simulink subsystem "Load"  (R2020b)
settings: Solver=VariableStepAuto  StartTime=0.0  StopTime=10.0  RelTol=1e-3
undefined symbols (not defined in the file): DCHigh, DCLow
libraries: nesl_utility x5, fl_lib x5
settings Model: Creator=cao2851  LastModifiedBy=cao2851
settings SimscapeCC: SimscapeNormalizeSystem=off

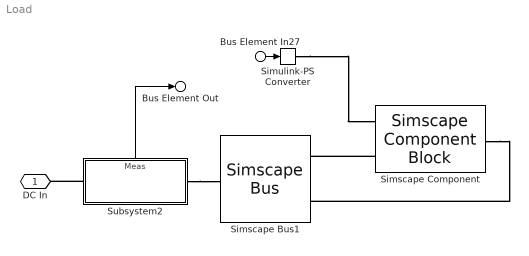
== system Load ==
  Bus Element In27 : Inport  PortName=Ctrl  Element=LoadSetpoint
  Simscape Component : SimscapeComponentBlock  SourceFile=VariablePowerLoad  ComponentPath=VariablePowerLoad  ComponentVariants="[\"VariablePowerLoad\"]"  ComponentVariantNames="[\"VariablePowerLoad\"]"  ClassName=VariablePowerLoad  SchemaVersion=1  Vsoll=350  Slope=100  MinV=0.7  MaxV=1.2  i_specify=off  i_priority=None  i=0 A  i_nominal_specify=off  i_nominal_unit=A  i_nominal_value=1  v_specify=off  v_priority=None  v=0 V  v_nominal_specify=off  v_nominal_unit=V  v_nominal_value=1  Psoll_specify=off  Psoll_priority=None  Psoll=0 W  Psoll_nominal_specify=off  Psoll_nominal_unit=W  Psoll_nominal_value=1
      settings: CopyFcn=simscape.engine.sli.internal.componentblockcallback(gcbh,'COPY')  PreCopyFcn=simscape.engine.sli.internal.componentblockcallback(gcbh,'PRECOPY')  PreDeleteFcn=simscape.engine.sli.internal.componentblockcallback(gcbh,'PREDELETE')  InternalSimscapePortConfiguration="{\"Bottom\":[],\"Left\":[{\"id\":\"Power\",\"label\":\"P\",\"type\":\"input\"},{\"id\":\"p\",\"label\":\"+\",\"type\":\"foundation.electrical.electrical\"}],\"Right\":[{\"id\":\"n\",\"label\":\"-\",\"type\":\"foundation.electrical.electrical\"}],\"Top\":[]}"
      mask Type: Variable power load. It might be necesarry to use local simscape solver.
  Simscape Bus1 : SimscapeBus  HierarchyStrings=DCHigh;DCLow
  Simulink-PS Converter : nesl_utility/Simulink-PS Converter  PhysicalDomain=network_engine_domain  SubClassName=ps_input  LeftPortType=input  RightPortType=output  PseudoPeriodic=off  Frequencies=[]  NoiseDistribution=none  NoiseParameters=[]  Unit=1  AffineConversion=off  FilteringAndDerivatives=provide  SimscapeFilterOrder=1  InputFilterTimeConstant=0.001  UdotUserProvided=0
  Subsystem2 : Subsystem
      settings: PortSchema="{\"entries\":[{\"content\":{\"sides\":[{\"content\":{\"connectorIds\":[\"LConn1\"]},\"type\":\"ConnectorPlacement.EquallySpacedRectSide\",\"uuid\":\"6ceb37b8-2165-4d7d-a6fb-f279e2d82052\"},{\"content\":{\"connectorIds\":[\"RConn1\"],\"side\":\"RIGHT\"},\"type\":\"ConnectorPlacement.EquallySpacedRectSide\",\"uuid\":\"4155948b-55c4-4bcd-990d-59b1d009d707\"},{\"content\":{\"connectorIds\":[\"Out1\"],\"side\":\"TOP\"},\"type\":\"ConnectorPlacement.EquallySpacedRectSide\",\"uuid\":\"00a7b829-f817-4a9f-907b-0b6347f161bc\"},{\"content\":{\"connectorIds\":[],\"side\":\"HIDDEN\"},\"type\":\"ConnectorPlacement.EquallySpacedRectSide\",\"uuid\":\"9dcb8e64-3042-4cb3-a9ae-ca9509bc434a\"}]},\"type\":\"ConnectorPlacement.EquallySpacedConnector\",\"uuid\":\"80bcd14e-b03c-415a-a271-317cb15dab1c\"}],\"packageUris\":[\"http://schema.mathworks.com/mf0/Connector/R2020b\"],\"version\":\"1.0\"}"
  DC In : PMIOPort  Side=Left
  Bus Element Out : Outport  PortName=Meas  Element=Input
  wires:
  Bus Element In27/1 -> Simulink-PS Converter/1
  Subsystem2/1(Meas) -> Bus Element Out/1
  connections:
  Simulink-PS Converter/RConn1 -- Simscape Component/LConn1
  Simscape Component/LConn2 -- Simscape Bus1/LConn1
  Simscape Component/RConn1 -- Simscape Bus1/LConn2
  Subsystem2/LConn1 -- DC In/RConn1
  Subsystem2/RConn1 -- Simscape Bus1/RConn1

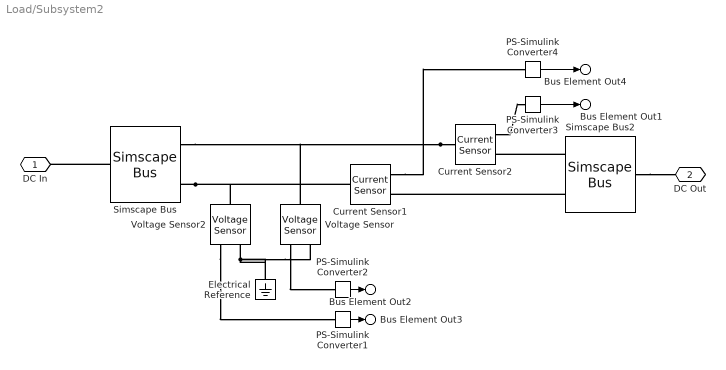
== system Load/Subsystem2 ==
  Current Sensor1 : fl_lib/Electrical/Electrical Sensors/Current Sensor
  Current Sensor2 : fl_lib/Electrical/Electrical Sensors/Current Sensor
  Electrical Reference : fl_lib/Electrical/Electrical Elements/Electrical Reference
  PS-Simulink Converter{1..4} (4 alike) : nesl_utility/PS-Simulink Converter  PhysicalDomain=network_engine_domain  SubClassName=ps_output  LeftPortType=input  RightPortType=output  PseudoPeriodic=off  Frequencies=[]  Unit=inherit  AffineConversion=off
      settings: SourceProductBaseCode=PW,SS
  Simscape Bus : SimscapeBus  HierarchyStrings=DCHigh;DCLow
  Simscape Bus2 : SimscapeBus  HierarchyStrings=DCHigh;DCLow
  Voltage Sensor : fl_lib/Electrical/Electrical Sensors/Voltage Sensor
  Voltage Sensor2 : fl_lib/Electrical/Electrical Sensors/Voltage Sensor
  DC In : PMIOPort  Side=Left
  DC Out : PMIOPort  Port=2  Side=Right
  Bus Element Out4 : Outport  PortName=Meas  Element=ILow
  Bus Element Out1 : Outport  PortName=Meas  Element=IHigh
  Bus Element Out3 : Outport  PortName=Meas  Element=VLow
  Bus Element Out2 : Outport  PortName=Meas  Element=VHigh
  wires:
  PS-Simulink Converter3/1 -> Bus Element Out1/1
  PS-Simulink Converter2/1 -> Bus Element Out2/1
  PS-Simulink Converter1/1 -> Bus Element Out3/1
  PS-Simulink Converter4/1 -> Bus Element Out4/1
  connections:
  Voltage Sensor2/RConn1 -- PS-Simulink Converter1/LConn1
  Simscape Bus2/LConn2 -- Current Sensor1/RConn2
  Simscape Bus2/LConn1 -- Current Sensor2/RConn2
  Current Sensor1/RConn1 -- PS-Simulink Converter4/LConn1
  Simscape Bus2/RConn1 -- DC Out/RConn1
  Voltage Sensor/RConn1 -- PS-Simulink Converter2/LConn1
  Simscape Bus/RConn1 -- DC In/RConn1
  Current Sensor2/RConn1 -- PS-Simulink Converter3/LConn1
  Simscape Bus/LConn2 -- Current Sensor1/LConn1 -- Voltage Sensor2/LConn1
  Current Sensor2/LConn1 -- Simscape Bus/LConn1 -- Voltage Sensor/LConn1
  Voltage Sensor2/RConn2 -- Voltage Sensor/RConn2 -- Electrical Reference/LConn1
